simulink model "MavicModel"  (R2020b)
settings: Solver=VariableStepAuto  StartTime=0.0  StopTime=100  RelTol=1e-3
libraries: pid_lib x6
settings Model: Creator=surya  LastModifiedBy=surya
settings SolverCC: ZeroCrossAlgorithm=Adaptive
settings DebuggingCC: IgnoredZcDiagnostic=none

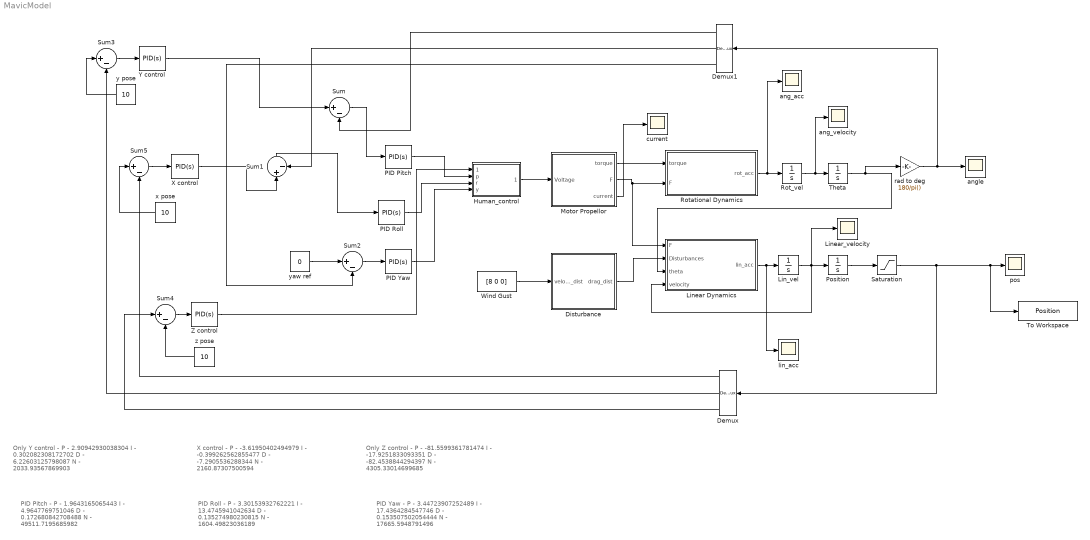
== system MavicModel ==
  note: PID Pitch -  P - 1.9643165065443
      | I - 4.9647769751046
      | D - 0.172680842708488
      | N - 49511.7195685982
  note: X control - P - -3.61950402494979
      | 	I - -0.399262562855477
      | 	D - 	-7.2905536288344
      | 	N - 2160.87307500594
  note: Only Z control - P  - -81.5599361781474
      | 			I  - -17.9251833093351
      | 			D  - -82.4538844294397
      | 			N  - 4305.33014699685
  note: Only Y control - P  - 2.90942930038304
      | 			I  -  0.302082308172702
      | 			D  -  6.22603125798087
      | 			N  -  2033.93567869903
  note: PID Roll - P - 3.30153932762221
      | I - 13.4745941042634
      | D - 0.135274980230815
      | N - 1604.49823036189
  note: PID Yaw - P - 3.44723907252489
      | I - 17.4364284547746
      | D - 0.153507502054444
      | N - 17665.5948791496
  " x pose" : Constant  Value=10
  " y pose" : Constant  Value=10
  " yaw ref" : Constant  Value=0
  " z pose" : Constant  Value=10
  Demux : Demux  Outputs=3
  Demux1 : Demux  Outputs=3
  Disturbance : MATLAB Function  TreatAsAtomicUnit=on
  Human_control : MATLAB Function  TreatAsAtomicUnit=on
  Lin_vel : Integrator
  Linear Dynamics : MATLAB Function  TreatAsAtomicUnit=on
  Linear_velocity : Scope
  Motor Propellor : MATLAB Function  TreatAsAtomicUnit=on
  PID Pitch : pid_lib/PID Controller  Controller=PID  Form=Parallel  TimeDomain=Continuous-time  UseExternalTs=off  SampleTime=-1  IntegratorMethod=Forward Euler  FilterMethod=Forward Euler  ControllerParametersSource=internal  P=1.9643165065443  I=4.9647769751046  D=0.172680842708488  UseFilter=on  N=49511.7195685982  TunerSelectOption=Transfer Function Based (PID Tuner App)  InitialConditionSource=internal  InitialConditionForIntegrator=0  InitialConditionForFilter=0  DifferentiatorICPrevScaledInput=0  ExternalReset=none  TrackingMode=off  Kt=1  LimitOutput=on  SatLimitsSource=internal  UpperSaturationLimit=50  LowerSaturationLimit=-50  LinearizeAsGain=on  AntiWindupMode=clamping  Kb=1  POutMin=[]  POutMax=[]  IOutMin=[]  IOutMax=[]  DOutMin=[]  DOutMax=[]  NOutMin=[]  NOutMax=[]  SumOutMin=[]  SumOutMax=[]  SaturationOutMin=[]  SaturationOutMax=[]  PParamMin=[]  PParamMax=[]  IParamMin=[]  IParamMax=[]  DParamMin=[]  DParamMax=[]  NParamMin=[]  NParamMax=[]  KbParamMin=[]  KbParamMax=[]  KtParamMin=[]  KtParamMax=[]  KbOutMin=[]  KbOutMax=[]  KtOutMin=[]  KtOutMax=[]  IntegratorOutMin=[]  IntegratorOutMax=[]  FilterOutMin=[]  FilterOutMax=[]  SumI1OutMin=[]  SumI1OutMax=[]  SumI2OutMin=[]  SumI2OutMax=[]  SumI3OutMin=[]  SumI3OutMax=[]  SumI4OutMin=[]  SumI4OutMax=[]  SumDOutMin=[]  SumDOutMax=[]  DifferentiatorOutMin=[]  DifferentiatorOutMax=[]  FilterDiffOutCoefMin=[]  FilterDiffOutCoefMax=[]  ReciprocalOutMin=[]  ReciprocalOutMax=[]  SumDenOutMin=[]  SumDenOutMax=[]  SumNumOutMin=[]  SumNumOutMax=[]  DivideOutMin=[]  DivideOutMax=[]  UdiffTsProdOutMin=[]  UdiffTsProdOutMax=[]  NTsProdOutMin=[]  NTsProdOutMax=[]  UintegralTsProdOutMin=[]  UintegralTsProdOutMax=[]  UngainTsProdOutMin=[]  UngainTsProdOutMax=[]  IntegratorContinuousStateAttributes=''  IntegratorStateMustResolveToSignalObject=off  IntegratorRTWStateStorageClass=Auto  FilterContinuousStateAttributes=''  FilterStateMustResolveToSignalObject=off  FilterRTWStateStorageClass=Auto  ParallelPVariant=InternalParameters  IdealPVariant=Disabled  IVariant=InternalParameters  DVariant=InternalParameters  IntegratorVariant=Continuous  SatVariant=Enabled  AWVariant=ContClampingParallel  PCopyVariant=Disabled  TRVariant=Disabled  FdbkBlocksVariant=Forward  IdealPFdbkVariant=Disabled  SatFdbkVariant=Disabled  DerivativeFilterVariant=ContFilter  NVariant=InternalParameters  NCopyVariant=Disabled  FilterICVariant=InternalICsFilter  IntegratorICVariant=InternalICs  ExternalResetVariant=Disabled  TRSumVariant=Passthrough  SumFdbkVariant=Disabled  SumVariant=Sum_PID  TsampFilterVariant=InternalTs  TsampNgainVariant=Passthrough  TsampIntegralVariant=Passthrough  ExternalSaturationOutDataTypeStr=Inherit: Same as second input
  PID Roll : pid_lib/PID Controller  Controller=PID  Form=Parallel  TimeDomain=Continuous-time  UseExternalTs=off  SampleTime=-1  IntegratorMethod=Forward Euler  FilterMethod=Forward Euler  ControllerParametersSource=internal  P=3.30153932762221  I=13.4745941042634  D=0.135274980230815  UseFilter=on  N=1604.49823036189  TunerSelectOption=Transfer Function Based (PID Tuner App)  InitialConditionSource=internal  InitialConditionForIntegrator=0  InitialConditionForFilter=0  DifferentiatorICPrevScaledInput=0  ExternalReset=none  TrackingMode=off  Kt=1  LimitOutput=on  SatLimitsSource=internal  UpperSaturationLimit=15  LowerSaturationLimit=-15  LinearizeAsGain=on  AntiWindupMode=clamping  Kb=1  POutMin=[]  POutMax=[]  IOutMin=[]  IOutMax=[]  DOutMin=[]  DOutMax=[]  NOutMin=[]  NOutMax=[]  SumOutMin=[]  SumOutMax=[]  SaturationOutMin=[]  SaturationOutMax=[]  PParamMin=[]  PParamMax=[]  IParamMin=[]  IParamMax=[]  DParamMin=[]  DParamMax=[]  NParamMin=[]  NParamMax=[]  KbParamMin=[]  KbParamMax=[]  KtParamMin=[]  KtParamMax=[]  KbOutMin=[]  KbOutMax=[]  KtOutMin=[]  KtOutMax=[]  IntegratorOutMin=[]  IntegratorOutMax=[]  FilterOutMin=[]  FilterOutMax=[]  SumI1OutMin=[]  SumI1OutMax=[]  SumI2OutMin=[]  SumI2OutMax=[]  SumI3OutMin=[]  SumI3OutMax=[]  SumI4OutMin=[]  SumI4OutMax=[]  SumDOutMin=[]  SumDOutMax=[]  DifferentiatorOutMin=[]  DifferentiatorOutMax=[]  FilterDiffOutCoefMin=[]  FilterDiffOutCoefMax=[]  ReciprocalOutMin=[]  ReciprocalOutMax=[]  SumDenOutMin=[]  SumDenOutMax=[]  SumNumOutMin=[]  SumNumOutMax=[]  DivideOutMin=[]  DivideOutMax=[]  UdiffTsProdOutMin=[]  UdiffTsProdOutMax=[]  NTsProdOutMin=[]  NTsProdOutMax=[]  UintegralTsProdOutMin=[]  UintegralTsProdOutMax=[]  UngainTsProdOutMin=[]  UngainTsProdOutMax=[]  IntegratorContinuousStateAttributes=''  IntegratorStateMustResolveToSignalObject=off  IntegratorRTWStateStorageClass=Auto  FilterContinuousStateAttributes=''  FilterStateMustResolveToSignalObject=off  FilterRTWStateStorageClass=Auto  ParallelPVariant=InternalParameters  IdealPVariant=Disabled  IVariant=InternalParameters  DVariant=InternalParameters  IntegratorVariant=Continuous  SatVariant=Enabled  AWVariant=ContClampingParallel  PCopyVariant=Disabled  TRVariant=Disabled  FdbkBlocksVariant=Forward  IdealPFdbkVariant=Disabled  SatFdbkVariant=Disabled  DerivativeFilterVariant=ContFilter  NVariant=InternalParameters  NCopyVariant=Disabled  FilterICVariant=InternalICsFilter  IntegratorICVariant=InternalICs  ExternalResetVariant=Disabled  TRSumVariant=Passthrough  SumFdbkVariant=Disabled  SumVariant=Sum_PID  TsampFilterVariant=InternalTs  TsampNgainVariant=Passthrough  TsampIntegralVariant=Passthrough  ExternalSaturationOutDataTypeStr=Inherit: Same as second input
  PID Yaw : pid_lib/PID Controller  Controller=PID  Form=Parallel  TimeDomain=Continuous-time  UseExternalTs=off  SampleTime=-1  IntegratorMethod=Forward Euler  FilterMethod=Forward Euler  ControllerParametersSource=internal  P=3.44723907252489  I=17.4364284547746  D=0.153507502054444  UseFilter=on  N=17665.5948791496  TunerSelectOption=Transfer Function Based (PID Tuner App)  InitialConditionSource=internal  InitialConditionForIntegrator=0  InitialConditionForFilter=0  DifferentiatorICPrevScaledInput=0  ExternalReset=none  TrackingMode=off  Kt=1  LimitOutput=on  SatLimitsSource=internal  UpperSaturationLimit=30  LowerSaturationLimit=-30  LinearizeAsGain=on  AntiWindupMode=clamping  Kb=1  POutMin=[]  POutMax=[]  IOutMin=[]  IOutMax=[]  DOutMin=[]  DOutMax=[]  NOutMin=[]  NOutMax=[]  SumOutMin=[]  SumOutMax=[]  SaturationOutMin=[]  SaturationOutMax=[]  PParamMin=[]  PParamMax=[]  IParamMin=[]  IParamMax=[]  DParamMin=[]  DParamMax=[]  NParamMin=[]  NParamMax=[]  KbParamMin=[]  KbParamMax=[]  KtParamMin=[]  KtParamMax=[]  KbOutMin=[]  KbOutMax=[]  KtOutMin=[]  KtOutMax=[]  IntegratorOutMin=[]  IntegratorOutMax=[]  FilterOutMin=[]  FilterOutMax=[]  SumI1OutMin=[]  SumI1OutMax=[]  SumI2OutMin=[]  SumI2OutMax=[]  SumI3OutMin=[]  SumI3OutMax=[]  SumI4OutMin=[]  SumI4OutMax=[]  SumDOutMin=[]  SumDOutMax=[]  DifferentiatorOutMin=[]  DifferentiatorOutMax=[]  FilterDiffOutCoefMin=[]  FilterDiffOutCoefMax=[]  ReciprocalOutMin=[]  ReciprocalOutMax=[]  SumDenOutMin=[]  SumDenOutMax=[]  SumNumOutMin=[]  SumNumOutMax=[]  DivideOutMin=[]  DivideOutMax=[]  UdiffTsProdOutMin=[]  UdiffTsProdOutMax=[]  NTsProdOutMin=[]  NTsProdOutMax=[]  UintegralTsProdOutMin=[]  UintegralTsProdOutMax=[]  UngainTsProdOutMin=[]  UngainTsProdOutMax=[]  IntegratorContinuousStateAttributes=''  IntegratorStateMustResolveToSignalObject=off  IntegratorRTWStateStorageClass=Auto  FilterContinuousStateAttributes=''  FilterStateMustResolveToSignalObject=off  FilterRTWStateStorageClass=Auto  ParallelPVariant=InternalParameters  IdealPVariant=Disabled  IVariant=InternalParameters  DVariant=InternalParameters  IntegratorVariant=Continuous  SatVariant=Enabled  AWVariant=ContClampingParallel  PCopyVariant=Disabled  TRVariant=Disabled  FdbkBlocksVariant=Forward  IdealPFdbkVariant=Disabled  SatFdbkVariant=Disabled  DerivativeFilterVariant=ContFilter  NVariant=InternalParameters  NCopyVariant=Disabled  FilterICVariant=InternalICsFilter  IntegratorICVariant=InternalICs  ExternalResetVariant=Disabled  TRSumVariant=Passthrough  SumFdbkVariant=Disabled  SumVariant=Sum_PID  TsampFilterVariant=InternalTs  TsampNgainVariant=Passthrough  TsampIntegralVariant=Passthrough  ExternalSaturationOutDataTypeStr=Inherit: Same as second input
  Position : Integrator
  Rot_vel : Integrator
  Rotational Dynamics : MATLAB Function  TreatAsAtomicUnit=on
  Saturation : Saturate  UpperLimit=inf  LowerLimit=[-inf,-inf,0]
  Sum{,1..5} (6 alike) : Sum  Inputs=|+-
  Theta : Integrator
  To Workspace : ToWorkspace  VariableName=Position  SampleTime=-1
      settings: Save2DSignal=2-D array (concatenate along first dimension)
  Wind Gust : Constant  Value=[8 0 0]
  X control : pid_lib/PID Controller  Controller=PID  Form=Parallel  TimeDomain=Continuous-time  UseExternalTs=off  SampleTime=-1  IntegratorMethod=Forward Euler  FilterMethod=Forward Euler  ControllerParametersSource=internal  P=-3.61950402494979  I=-0.399262562855477  D=-7.2905536288344  UseFilter=on  N=2160.87307500594  TunerSelectOption=Transfer Function Based (PID Tuner App)  InitialConditionSource=internal  InitialConditionForIntegrator=0  InitialConditionForFilter=0  DifferentiatorICPrevScaledInput=0  ExternalReset=none  TrackingMode=off  Kt=1  LimitOutput=on  SatLimitsSource=internal  UpperSaturationLimit=20  LowerSaturationLimit=-20  LinearizeAsGain=on  AntiWindupMode=clamping  Kb=1  POutMin=[]  POutMax=[]  IOutMin=[]  IOutMax=[]  DOutMin=[]  DOutMax=[]  NOutMin=[]  NOutMax=[]  SumOutMin=[]  SumOutMax=[]  SaturationOutMin=[]  SaturationOutMax=[]  PParamMin=[]  PParamMax=[]  IParamMin=[]  IParamMax=[]  DParamMin=[]  DParamMax=[]  NParamMin=[]  NParamMax=[]  KbParamMin=[]  KbParamMax=[]  KtParamMin=[]  KtParamMax=[]  KbOutMin=[]  KbOutMax=[]  KtOutMin=[]  KtOutMax=[]  IntegratorOutMin=[]  IntegratorOutMax=[]  FilterOutMin=[]  FilterOutMax=[]  SumI1OutMin=[]  SumI1OutMax=[]  SumI2OutMin=[]  SumI2OutMax=[]  SumI3OutMin=[]  SumI3OutMax=[]  SumI4OutMin=[]  SumI4OutMax=[]  SumDOutMin=[]  SumDOutMax=[]  DifferentiatorOutMin=[]  DifferentiatorOutMax=[]  FilterDiffOutCoefMin=[]  FilterDiffOutCoefMax=[]  ReciprocalOutMin=[]  ReciprocalOutMax=[]  SumDenOutMin=[]  SumDenOutMax=[]  SumNumOutMin=[]  SumNumOutMax=[]  DivideOutMin=[]  DivideOutMax=[]  UdiffTsProdOutMin=[]  UdiffTsProdOutMax=[]  NTsProdOutMin=[]  NTsProdOutMax=[]  UintegralTsProdOutMin=[]  UintegralTsProdOutMax=[]  UngainTsProdOutMin=[]  UngainTsProdOutMax=[]  IntegratorContinuousStateAttributes=''  IntegratorStateMustResolveToSignalObject=off  IntegratorRTWStateStorageClass=Auto  FilterContinuousStateAttributes=''  FilterStateMustResolveToSignalObject=off  FilterRTWStateStorageClass=Auto  ParallelPVariant=InternalParameters  IdealPVariant=Disabled  IVariant=InternalParameters  DVariant=InternalParameters  IntegratorVariant=Continuous  SatVariant=Enabled  AWVariant=ContClampingParallel  PCopyVariant=Disabled  TRVariant=Disabled  FdbkBlocksVariant=Forward  IdealPFdbkVariant=Disabled  SatFdbkVariant=Disabled  DerivativeFilterVariant=ContFilter  NVariant=InternalParameters  NCopyVariant=Disabled  FilterICVariant=InternalICsFilter  IntegratorICVariant=InternalICs  ExternalResetVariant=Disabled  TRSumVariant=Passthrough  SumFdbkVariant=Disabled  SumVariant=Sum_PID  TsampFilterVariant=InternalTs  TsampNgainVariant=Passthrough  TsampIntegralVariant=Passthrough  ExternalSaturationOutDataTypeStr=Inherit: Same as second input
  Y control : pid_lib/PID Controller  Controller=PID  Form=Parallel  TimeDomain=Continuous-time  UseExternalTs=off  SampleTime=-1  IntegratorMethod=Forward Euler  FilterMethod=Forward Euler  ControllerParametersSource=internal  P=2.90942930038304  I=0.302082308172702  D=6.22603125798087  UseFilter=on  N=2033.93567869903  TunerSelectOption=Transfer Function Based (PID Tuner App)  InitialConditionSource=internal  InitialConditionForIntegrator=0  InitialConditionForFilter=0  DifferentiatorICPrevScaledInput=0  ExternalReset=none  TrackingMode=off  Kt=1  LimitOutput=on  SatLimitsSource=internal  UpperSaturationLimit=20  LowerSaturationLimit=-20  LinearizeAsGain=on  AntiWindupMode=none  Kb=1  POutMin=[]  POutMax=[]  IOutMin=[]  IOutMax=[]  DOutMin=[]  DOutMax=[]  NOutMin=[]  NOutMax=[]  SumOutMin=[]  SumOutMax=[]  SaturationOutMin=[]  SaturationOutMax=[]  PParamMin=[]  PParamMax=[]  IParamMin=[]  IParamMax=[]  DParamMin=[]  DParamMax=[]  NParamMin=[]  NParamMax=[]  KbParamMin=[]  KbParamMax=[]  KtParamMin=[]  KtParamMax=[]  KbOutMin=[]  KbOutMax=[]  KtOutMin=[]  KtOutMax=[]  IntegratorOutMin=[]  IntegratorOutMax=[]  FilterOutMin=[]  FilterOutMax=[]  SumI1OutMin=[]  SumI1OutMax=[]  SumI2OutMin=[]  SumI2OutMax=[]  SumI3OutMin=[]  SumI3OutMax=[]  SumI4OutMin=[]  SumI4OutMax=[]  SumDOutMin=[]  SumDOutMax=[]  DifferentiatorOutMin=[]  DifferentiatorOutMax=[]  FilterDiffOutCoefMin=[]  FilterDiffOutCoefMax=[]  ReciprocalOutMin=[]  ReciprocalOutMax=[]  SumDenOutMin=[]  SumDenOutMax=[]  SumNumOutMin=[]  SumNumOutMax=[]  DivideOutMin=[]  DivideOutMax=[]  UdiffTsProdOutMin=[]  UdiffTsProdOutMax=[]  NTsProdOutMin=[]  NTsProdOutMax=[]  UintegralTsProdOutMin=[]  UintegralTsProdOutMax=[]  UngainTsProdOutMin=[]  UngainTsProdOutMax=[]  IntegratorContinuousStateAttributes=''  IntegratorStateMustResolveToSignalObject=off  IntegratorRTWStateStorageClass=Auto  FilterContinuousStateAttributes=''  FilterStateMustResolveToSignalObject=off  FilterRTWStateStorageClass=Auto  ParallelPVariant=InternalParameters  IdealPVariant=Disabled  IVariant=InternalParameters  DVariant=InternalParameters  IntegratorVariant=Continuous  SatVariant=Enabled  AWVariant=Passthrough  PCopyVariant=Disabled  TRVariant=Disabled  FdbkBlocksVariant=Forward  IdealPFdbkVariant=Disabled  SatFdbkVariant=Disabled  DerivativeFilterVariant=ContFilter  NVariant=InternalParameters  NCopyVariant=Disabled  FilterICVariant=InternalICsFilter  IntegratorICVariant=InternalICs  ExternalResetVariant=Disabled  TRSumVariant=Passthrough  SumFdbkVariant=Disabled  SumVariant=Sum_PID  TsampFilterVariant=InternalTs  TsampNgainVariant=Passthrough  TsampIntegralVariant=Passthrough  ExternalSaturationOutDataTypeStr=Inherit: Same as second input
  Z control : pid_lib/PID Controller  Controller=PID  Form=Parallel  TimeDomain=Continuous-time  UseExternalTs=off  SampleTime=-1  IntegratorMethod=Forward Euler  FilterMethod=Forward Euler  ControllerParametersSource=internal  P=-81.5599361781474  I=-17.9251833093351  D=-82.4538844294397  UseFilter=on  N=4305.33014699685  TunerSelectOption=Transfer Function Based (PID Tuner App)  InitialConditionSource=internal  InitialConditionForIntegrator=0  InitialConditionForFilter=0  DifferentiatorICPrevScaledInput=0  ExternalReset=none  TrackingMode=off  Kt=1  LimitOutput=on  SatLimitsSource=internal  UpperSaturationLimit=100  LowerSaturationLimit=20  LinearizeAsGain=on  AntiWindupMode=none  Kb=1  POutMin=[]  POutMax=[]  IOutMin=[]  IOutMax=[]  DOutMin=[]  DOutMax=[]  NOutMin=[]  NOutMax=[]  SumOutMin=[]  SumOutMax=[]  SaturationOutMin=[]  SaturationOutMax=[]  PParamMin=[]  PParamMax=[]  IParamMin=[]  IParamMax=[]  DParamMin=[]  DParamMax=[]  NParamMin=[]  NParamMax=[]  KbParamMin=[]  KbParamMax=[]  KtParamMin=[]  KtParamMax=[]  KbOutMin=[]  KbOutMax=[]  KtOutMin=[]  KtOutMax=[]  IntegratorOutMin=[]  IntegratorOutMax=[]  FilterOutMin=[]  FilterOutMax=[]  SumI1OutMin=[]  SumI1OutMax=[]  SumI2OutMin=[]  SumI2OutMax=[]  SumI3OutMin=[]  SumI3OutMax=[]  SumI4OutMin=[]  SumI4OutMax=[]  SumDOutMin=[]  SumDOutMax=[]  DifferentiatorOutMin=[]  DifferentiatorOutMax=[]  FilterDiffOutCoefMin=[]  FilterDiffOutCoefMax=[]  ReciprocalOutMin=[]  ReciprocalOutMax=[]  SumDenOutMin=[]  SumDenOutMax=[]  SumNumOutMin=[]  SumNumOutMax=[]  DivideOutMin=[]  DivideOutMax=[]  UdiffTsProdOutMin=[]  UdiffTsProdOutMax=[]  NTsProdOutMin=[]  NTsProdOutMax=[]  UintegralTsProdOutMin=[]  UintegralTsProdOutMax=[]  UngainTsProdOutMin=[]  UngainTsProdOutMax=[]  IntegratorContinuousStateAttributes=''  IntegratorStateMustResolveToSignalObject=off  IntegratorRTWStateStorageClass=Auto  FilterContinuousStateAttributes=''  FilterStateMustResolveToSignalObject=off  FilterRTWStateStorageClass=Auto  ParallelPVariant=InternalParameters  IdealPVariant=Disabled  IVariant=InternalParameters  DVariant=InternalParameters  IntegratorVariant=Continuous  SatVariant=Enabled  AWVariant=Passthrough  PCopyVariant=Disabled  TRVariant=Disabled  FdbkBlocksVariant=Forward  IdealPFdbkVariant=Disabled  SatFdbkVariant=Disabled  DerivativeFilterVariant=ContFilter  NVariant=InternalParameters  NCopyVariant=Disabled  FilterICVariant=InternalICsFilter  IntegratorICVariant=InternalICs  ExternalResetVariant=Disabled  TRSumVariant=Passthrough  SumFdbkVariant=Disabled  SumVariant=Sum_PID  TsampFilterVariant=InternalTs  TsampNgainVariant=Passthrough  TsampIntegralVariant=Passthrough  ExternalSaturationOutDataTypeStr=Inherit: Same as second input
  ang_acc : Scope
  ang_velocity : Scope
  angle : Scope
  current : Scope
  lin_acc : Scope
  pos : Scope
  rad to deg : Gain  Gain=180/pi()
  wires:
  Motor Propellor/1(torque) -> Rotational Dynamics/1(torque)
  Motor Propellor/2(F) -> Linear Dynamics/1(F), Rotational Dynamics/2(F)
  Rotational Dynamics/1(rot_acc) -> ang_acc/1, Rot_vel/1
  Theta/1 -> rad to deg/1, Linear Dynamics/3(theta)
  Linear Dynamics/1(lin_acc) -> lin_acc/1, Lin_vel/1
  Lin_vel/1 -> Position/1, Linear_velocity/1, Linear Dynamics/4(velocity)
  Disturbance/1(drag_dist) -> Linear Dynamics/2(Disturbances)
  Wind Gust/1 -> Disturbance/1(velocity_dist)
  Human_control/1(voltage) -> Motor Propellor/1(Voltage)
  rad to deg/1 -> Demux1/1, angle/1
  Motor Propellor/3(current) -> current/1
  Sum/1 -> PID Pitch/1
  PID Pitch/1 -> Human_control/2(p)
  Demux1/1 -> Sum/2
  PID Roll/1 -> Human_control/3(r)
  Sum1/1 -> PID Roll/1
  Demux1/2 -> Sum1/2
  Sum2/1 -> PID Yaw/1
  PID Yaw/1 -> Human_control/4(y)
  Rot_vel/1 -> ang_velocity/1, Theta/1
  Position/1 -> Saturation/1
  Saturation/1 -> Demux/1, pos/1, To Workspace/1
  Sum3/1 -> Y control/1
  Demux/2 -> Sum3/2
  " y pose"/1 -> Sum3/1
  Y control/1 -> Sum/1
  Demux/1 -> Sum5/2
  Sum5/1 -> X control/1
  " x pose"/1 -> Sum5/1
  Sum4/1 -> Z control/1
  Demux/3 -> Sum4/1
  " z pose"/1 -> Sum4/2
  Z control/1 -> Human_control/1(throttle)
  Demux1/3 -> Sum2/2
  " yaw ref"/1 -> Sum2/1
  X control/1 -> Sum1/1

== matlab function MavicModel/Rotational Dynamics ==
  data: torque input; rot_acc output; F input
function rot_acc = fcn(torque, F)
Moment = [0, 0, 0];  %x y z axis moments
rot_acc = [0, 0, 0];  %x y z rot_acceleration
I = [0.003, 0.003, 0.007];  %Moment of inertia about x y z axis
Moment(1) = (F(3) + F(4))*0.237/2 - (F(1) + F(2))*0.237/2;   % +ve - pitch forward
Moment(2) = (F(2) + F(3))*0.237/2 - (F(1) + F(4))*0.237/2;   % +ve - roll clockwise from front
Moment(3) = -(torque(4) + torque(2) + torque(1) + torque(3)); % +ve - yaw clockwise from top
for i=1:3
    rot_acc(i) = Moment(i)/I(i);
end
end

== matlab function MavicModel/Motor Propellor ==
  data: Voltage input; torque output; F output; current output
function [torque, F, current] = fcn(Voltage)
RPM = [0, 0, 0, 0];
torque = [0, 0, 0, 0];
current = [0, 0, 0, 0];
F=[0, 0, 0, 0];
K_v = 1400;

RPM = 2.6931*Voltage.^3+1400*Voltage;
Ct = 2*10^-15*RPM.^3-4*10^-11*RPM.^2+3*10^-7*RPM+0.1013;
F = Ct*1.225.*(RPM/60).^2*(0.2)^4;
for i=1:4    
    torque(i) = -(-1)^(i)*(4*10^-14*RPM(i)^3 + 8*10^-12*RPM(i)^2 + 3*10^-6*RPM(i));
    current(i) = K_v * torque(i);
end
end

== matlab function MavicModel/Linear Dynamics ==
  data: F input; lin_acc output; Disturbances input; theta input; velocity input
function lin_acc = fcn(F, Disturbances, theta, velocity)
m = 0.743;  %Mass of drone
g = 9.81;  %Acc due to gravity
A = [0.0197, 0.0197, 0.0512];  %x y z Projected area
rho = 1.225;  %Density of air
Cd = 1.7; %Coeff of Drag

lin_acc = [0 0 0];
force = [0 0 0];
fprop = [0 0 0];

%% Roll and Pitch Thrust Vector
fprop(1) = -sin(theta(2))*cos(theta(1))*(F(1) + F(2) + F(3) + F(4));   % Prop force on body x axis
fprop(2) = sin(theta(1))*cos(theta(2))*(F(1) + F(2) + F(3) + F(4));   % Prop force on body y axis
fprop(3) = cos(theta(1))*cos(theta(2))*(F(1) + F(2) + F(3)+ F(4));  % Prop force on body z axis

%% Yaw Thrust Vector
thetaxy = atan2(fprop(1),fprop(2));  % radians  was -ve earlier
xy2D = sqrt(fprop(1)^2 + fprop(2)^2);
if fprop(3)>=0
    fprop(1) = xy2D*sin(thetaxy + theta(3));  % prop force on world x-axis
    fprop(2) = xy2D*cos(thetaxy + theta(3));  % prop force on world y-axis
else
    fprop(1) = xy2D*sin(thetaxy - theta(3));
    fprop(2) = xy2D*cos(thetaxy - theta(3));
end

if velocity(1)<0
    force(1) = fprop(1) - Disturbances(1) + 0.5*rho*velocity(1)^2*A(1)*Cd;
else
    force(1) = fprop(1) - Disturbances(1) - 0.5*rho*velocity(1)^2*A(1)*Cd;
end

if velocity(2)<0
    force(2) = fprop(2) - Disturbances(2) + 0.5*rho*velocity(2)^2*A(2)*Cd;
else
    force(2) = fprop(2) - Disturbances(2) - 0.5*rho*velocity(2)^2*A(2)*Cd;
end

if velocity(3)<0
    force(3) = fprop(3) - Disturbances(3) + 0.5*rho*velocity(3)^2*A(3)*Cd - m*g;
else
    force(3) = fprop(3) - Disturbances(3) - 0.5*rho*velocity(3)^2*A(3)*Cd - m*g;
end
%% Linear Acceleration

for i=1:3
    lin_acc(i) = force(i)/m;
end

== matlab function MavicModel/Disturbance ==
  data: velocity_dist input; drag_dist output
function drag_dist = fcn(velocity_dist)
A = [0.0197 0.0197 0.0197*2];
drag_dist = [0 0 0];
rho = 1.225;
Cd = 1;
for i=1:3
    drag_dist(i) = 0.5*rho*velocity_dist(i)^2*A(i)*Cd;
    if velocity_dist(i)>0   %Was greater earlier
        drag_dist(i) = -drag_dist(i);
    end
end

== matlab function MavicModel/Human_control ==
  data: throttle input; voltage output; p input; r input; y input
function voltage = fcn(throttle, p, r, y)
correct = 0;
if (p/2 + r/2 + y/2)>(100-throttle)
    correct = (p/2 + r/2 + y/2) - (100 - throttle);
end
if (p/2 + r/2 + y/2)>(throttle)
    if correct<((p/2 + r/2 + y/2)-(throttle))
        correct = (p/2 + r/2 + y/2) - (throttle);
    end
end

% if correct ~= 0 
%     if (p - correct/3*2) < 0
%         p = 0;
%     else
%         p = p - correct/3*2;
%     end
%     
%     if (r - correct/3*2) < 0
%         r = 0;
%     else
%         r = r - correct/3*2;
%     end
%     
%     if (y - correct/3*2) < 0
%         y = 0;
%     else
%         y = y - correct/3*2;
%     end
% end

if correct ~= 0
    p = p - correct/3*2;
    r = r - correct/3*2;
    y = y - correct/3*2;
end

if throttle == 0
    p=0;
    r=0;
    y=0;
end

voltage = [(throttle-p/2-r/2-y/2)*11.4/100, (throttle-p/2+r/2+y/2)*11.4/100, (throttle+p/2+r/2-y/2)*11.4/100, (throttle+p/2-r/2+y/2)*11.4/100];
